simulink model "imageSendExample1"  (R2014a)
settings: configuration reference "AR_Drone_ConfigSet" (kept outside this file)
undefined symbols (not defined in the file): Afilter, Afilterphi, Amat, Bd, KDphi, KDphi_adjust, KDpsic, KDtheta, KDtheta_adjust, KDxc, KDyc, KDzc, KPphi, KPphi_adjust, KPpsic, KPtheta, KPtheta_adjust, KPxc, KPyc, KPzc, L, LA, LAphi, m
libraries: simulink x8, dspmtrx3 x5, AR_Drone_2_Library x4, ARdrone_video_lib x4, dspstat3 x2
(part 2 of 2)

== system imageSendExample1/Navigation Subsystem/CheckSum Pre-Processing/TempFilter/CheckSum Correction ==
  CalculatedData : Inport
  CheckSumFlag : Inport  Port=2
  Holding Value : Inport  Port=3
  Compare To Zero : simulink/Logic and Bit Operations/Compare To Zero  relop=>  OutDataTypeStr=boolean
  Delay : Delay  DelayLength=3  InitialCondition=0
  Generate Sample Holding Pulse : Subsystem
  "If True, we have good data, If false, we have bad data, With bad data, use previous good data from N samples ago and hold it on that value for M samples" : Switch  Criteria=u2 > Threshold
  Invert Logic : Logic  Operator=NOT  AllPortsSameDT=off  OutDataTypeStr=boolean
  Logical Operator1 : Logic  Operator=NOT  AllPortsSameDT=off  OutDataTypeStr=boolean
  Pre-Processed Data : Outport
  wires:
  CheckSumFlag/1 -> Compare To Zero/1
  CalculatedData/1 -> "If True, we have good data, If false, we have bad data, With bad data, use previous good data from N samples ago and hold it on that value for M samples"/1
  "If True, we have good data, If false, we have bad data, With bad data, use previous good data from N samples ago and hold it on that value for M samples"/1 -> Pre-Processed Data/1, Delay/1
  Delay/1 -> "If True, we have good data, If false, we have bad data, With bad data, use previous good data from N samples ago and hold it on that value for M samples"/3
  Compare To Zero/1 -> Logical Operator1/1
  Generate Sample Holding Pulse/1(Hold_Data_Pulse) -> Invert Logic/1
  Logical Operator1/1 -> Generate Sample Holding Pulse/1(CheckSumFlag)
  Invert Logic/1 -> "If True, we have good data, If false, we have bad data, With bad data, use previous good data from N samples ago and hold it on that value for M samples"/2
  Holding Value/1 -> Generate Sample Holding Pulse/2(HoldDataTicks_Value)

== system imageSendExample1/Navigation Subsystem/CheckSum Pre-Processing/TempFilter/Process Raw Mag Data ==
  note: magnetometer[ 0 ] = - ( float ) navdata.mx ;
      | magnetometer[ 1 ] = ( float ) navdata.my ;
      | magnetometer[ 2 ] = - ( float ) navdata.mz ;
      | const float Sensitivity[ 3 ] = { 0.0071492608 , 0.0070882491 , 0.0074057781 } ;
      | const float Neutral[ 3 ] = { 118.0 , - 65.0 , 110.0 } ;
  Magnetometer : Inport
  Bias : Constant  Value=[ 118.0, -65.0, 110.0 ]
  Sum : Sum  Inputs=|+-
  postGain : Gain  Gain=[0.0071492608, 0.0070882491, 0.0074057781]
  preGain : Gain  Gain=[-1 1 -1]
  ProcessedData : Outport
  wires:
  postGain/1 -> ProcessedData/1
  Magnetometer/1 -> preGain/1
  Sum/1 -> postGain/1
  preGain/1 -> Sum/1
  Bias/1 -> Sum/2

== system imageSendExample1/Navigation Subsystem/CheckSum Pre-Processing/TempFilter1/CheckSum Correction ==
  CalculatedData : Inport
  CheckSumFlag : Inport  Port=2
  Holding Value : Inport  Port=3
  Compare To Zero : simulink/Logic and Bit Operations/Compare To Zero  relop=>  OutDataTypeStr=boolean
  Delay : Delay  DelayLength=3  InitialCondition=0
  Generate Sample Holding Pulse : Subsystem
  "If True, we have good data, If false, we have bad data, With bad data, use previous good data from N samples ago and hold it on that value for M samples" : Switch  Criteria=u2 > Threshold
  Invert Logic : Logic  Operator=NOT  AllPortsSameDT=off  OutDataTypeStr=boolean
  Logical Operator1 : Logic  Operator=NOT  AllPortsSameDT=off  OutDataTypeStr=boolean
  Pre-Processed Data : Outport
  wires:
  CheckSumFlag/1 -> Compare To Zero/1
  CalculatedData/1 -> "If True, we have good data, If false, we have bad data, With bad data, use previous good data from N samples ago and hold it on that value for M samples"/1
  "If True, we have good data, If false, we have bad data, With bad data, use previous good data from N samples ago and hold it on that value for M samples"/1 -> Pre-Processed Data/1, Delay/1
  Delay/1 -> "If True, we have good data, If false, we have bad data, With bad data, use previous good data from N samples ago and hold it on that value for M samples"/3
  Compare To Zero/1 -> Logical Operator1/1
  Generate Sample Holding Pulse/1(Hold_Data_Pulse) -> Invert Logic/1
  Logical Operator1/1 -> Generate Sample Holding Pulse/1(CheckSumFlag)
  Invert Logic/1 -> "If True, we have good data, If false, we have bad data, With bad data, use previous good data from N samples ago and hold it on that value for M samples"/2
  Holding Value/1 -> Generate Sample Holding Pulse/2(HoldDataTicks_Value)

== system imageSendExample1/Navigation Subsystem/CheckSum Pre-Processing/TempFilter1/Process Raw Mag Data ==
  note: magnetometer[ 0 ] = - ( float ) navdata.mx ;
      | magnetometer[ 1 ] = ( float ) navdata.my ;
      | magnetometer[ 2 ] = - ( float ) navdata.mz ;
      | const float Sensitivity[ 3 ] = { 0.0071492608 , 0.0070882491 , 0.0074057781 } ;
      | const float Neutral[ 3 ] = { 118.0 , - 65.0 , 110.0 } ;
  Magnetometer : Inport
  Bias : Constant  Value=[ 118.0, -65.0, 110.0 ]
  Sum : Sum  Inputs=|+-
  postGain : Gain  Gain=[0.0071492608, 0.0070882491, 0.0074057781]
  preGain : Gain  Gain=[-1 1 -1]
  ProcessedData : Outport
  wires:
  postGain/1 -> ProcessedData/1
  Magnetometer/1 -> preGain/1
  Sum/1 -> postGain/1
  preGain/1 -> Sum/1
  Bias/1 -> Sum/2

== system imageSendExample1/Navigation Subsystem/CheckSum Pre-Processing/Ultrasound Processing/CheckSum Correction ==
  CalculatedData : Inport
  CheckSumFlag : Inport  Port=2
  Holding Value : Inport  Port=3
  Compare To Zero : simulink/Logic and Bit Operations/Compare To Zero  relop=>  OutDataTypeStr=boolean
  Delay : Delay  DelayLength=3  InitialCondition=0
  Generate Sample Holding Pulse : Subsystem
  "If True, we have good data, If false, we have bad data, With bad data, use previous good data from N samples ago and hold it on that value for M samples" : Switch  Criteria=u2 > Threshold
  Invert Logic : Logic  Operator=NOT  AllPortsSameDT=off  OutDataTypeStr=boolean
  Logical Operator1 : Logic  Operator=NOT  AllPortsSameDT=off  OutDataTypeStr=boolean
  Pre-Processed Height : Outport
  wires:
  CheckSumFlag/1 -> Compare To Zero/1
  CalculatedData/1 -> "If True, we have good data, If false, we have bad data, With bad data, use previous good data from N samples ago and hold it on that value for M samples"/1
  "If True, we have good data, If false, we have bad data, With bad data, use previous good data from N samples ago and hold it on that value for M samples"/1 -> Pre-Processed Height/1, Delay/1
  Delay/1 -> "If True, we have good data, If false, we have bad data, With bad data, use previous good data from N samples ago and hold it on that value for M samples"/3
  Compare To Zero/1 -> Logical Operator1/1
  Generate Sample Holding Pulse/1(Hold_Data_Pulse) -> Invert Logic/1
  Logical Operator1/1 -> Generate Sample Holding Pulse/1(CheckSumFlag)
  Invert Logic/1 -> "If True, we have good data, If false, we have bad data, With bad data, use previous good data from N samples ago and hold it on that value for M samples"/2
  Holding Value/1 -> Generate Sample Holding Pulse/2(HoldDataTicks_Value)

== system imageSendExample1/Navigation Subsystem/CheckSum Pre-Processing/Accelerometer Processing/CheckSum Correction/Generate Sample Holding Pulse ==
  CheckSumFlag : Inport
  HoldDataTicks_Value : Inport  Port=2
  Chart : Stateflow chart  TreatAsAtomicUnit=on
  Constant2 : Constant
  Logical Operator1 : Logic  AllPortsSameDT=off  OutDataTypeStr=boolean
  Transition Logic Detection : Subsystem
  Hold_Data_Pulse : Outport
  wires:
  Constant2/1 -> Logical Operator1/1
  Logical Operator1/1 -> Hold_Data_Pulse/1
  Chart/1(output) -> Logical Operator1/2
  Transition Logic Detection/1(Transition Detect) -> Chart/1(if_transition)
  CheckSumFlag/1 -> Transition Logic Detection/1(Input)
  HoldDataTicks_Value/1 -> Chart/2(HoldDataTicks)

== system imageSendExample1/Navigation Subsystem/CheckSum Pre-Processing/Magnetometer/CheckSum Correction/Generate Sample Holding Pulse ==
  CheckSumFlag : Inport
  HoldDataTicks_Value : Inport  Port=2
  Chart : Stateflow chart  TreatAsAtomicUnit=on
  Constant2 : Constant
  Logical Operator1 : Logic  AllPortsSameDT=off  OutDataTypeStr=boolean
  Transition Logic Detection : Subsystem
  Hold_Data_Pulse : Outport
  wires:
  Constant2/1 -> Logical Operator1/1
  Logical Operator1/1 -> Hold_Data_Pulse/1
  Chart/1(output) -> Logical Operator1/2
  Transition Logic Detection/1(Transition Detect) -> Chart/1(if_transition)
  CheckSumFlag/1 -> Transition Logic Detection/1(Input)
  HoldDataTicks_Value/1 -> Chart/2(HoldDataTicks)

== system imageSendExample1/Navigation Subsystem/CheckSum Pre-Processing/RateGyro Processing/CheckSum Correction/Generate Sample Holding Pulse ==
  CheckSumFlag : Inport
  HoldDataTicks_Value : Inport  Port=2
  Chart : Stateflow chart  TreatAsAtomicUnit=on
  Constant2 : Constant
  Logical Operator1 : Logic  AllPortsSameDT=off  OutDataTypeStr=boolean
  Transition Logic Detection : Subsystem
  Hold_Data_Pulse : Outport
  wires:
  Constant2/1 -> Logical Operator1/1
  Logical Operator1/1 -> Hold_Data_Pulse/1
  Chart/1(output) -> Logical Operator1/2
  Transition Logic Detection/1(Transition Detect) -> Chart/1(if_transition)
  CheckSumFlag/1 -> Transition Logic Detection/1(Input)
  HoldDataTicks_Value/1 -> Chart/2(HoldDataTicks)

== system imageSendExample1/Navigation Subsystem/CheckSum Pre-Processing/TempFilter/CheckSum Correction/Generate Sample Holding Pulse ==
  CheckSumFlag : Inport
  HoldDataTicks_Value : Inport  Port=2
  Chart : Stateflow chart  TreatAsAtomicUnit=on
  Constant2 : Constant
  Logical Operator1 : Logic  AllPortsSameDT=off  OutDataTypeStr=boolean
  Transition Logic Detection : Subsystem
  Hold_Data_Pulse : Outport
  wires:
  Constant2/1 -> Logical Operator1/1
  Logical Operator1/1 -> Hold_Data_Pulse/1
  Chart/1(output) -> Logical Operator1/2
  Transition Logic Detection/1(Transition Detect) -> Chart/1(if_transition)
  CheckSumFlag/1 -> Transition Logic Detection/1(Input)
  HoldDataTicks_Value/1 -> Chart/2(HoldDataTicks)

== system imageSendExample1/Navigation Subsystem/CheckSum Pre-Processing/TempFilter1/CheckSum Correction/Generate Sample Holding Pulse ==
  CheckSumFlag : Inport
  HoldDataTicks_Value : Inport  Port=2
  Chart : Stateflow chart  TreatAsAtomicUnit=on
  Constant2 : Constant
  Logical Operator1 : Logic  AllPortsSameDT=off  OutDataTypeStr=boolean
  Transition Logic Detection : Subsystem
  Hold_Data_Pulse : Outport
  wires:
  Constant2/1 -> Logical Operator1/1
  Logical Operator1/1 -> Hold_Data_Pulse/1
  Chart/1(output) -> Logical Operator1/2
  Transition Logic Detection/1(Transition Detect) -> Chart/1(if_transition)
  CheckSumFlag/1 -> Transition Logic Detection/1(Input)
  HoldDataTicks_Value/1 -> Chart/2(HoldDataTicks)

== system imageSendExample1/Navigation Subsystem/CheckSum Pre-Processing/Ultrasound Processing/CheckSum Correction/Generate Sample Holding Pulse ==
  CheckSumFlag : Inport
  HoldDataTicks_Value : Inport  Port=2
  Chart : Stateflow chart  TreatAsAtomicUnit=on
  Constant2 : Constant
  Logical Operator1 : Logic  AllPortsSameDT=off  OutDataTypeStr=boolean
  Transition Logic Detection : Subsystem
  Hold_Data_Pulse : Outport
  wires:
  Constant2/1 -> Logical Operator1/1
  Logical Operator1/1 -> Hold_Data_Pulse/1
  Chart/1(output) -> Logical Operator1/2
  Transition Logic Detection/1(Transition Detect) -> Chart/1(if_transition)
  CheckSumFlag/1 -> Transition Logic Detection/1(Input)
  HoldDataTicks_Value/1 -> Chart/2(HoldDataTicks)

== system imageSendExample1/Navigation Subsystem/CheckSum Pre-Processing/Accelerometer Processing/CheckSum Correction/Generate Sample Holding Pulse/Transition Logic Detection ==
  Input : Inport
  Constant : Constant  Value=0
  Constant1 : Constant
  Logical Operator : Logic  AllPortsSameDT=off  OutDataTypeStr=boolean
  Relational Operator : RelationalOperator  Operator===  OutDataTypeStr=boolean
  Relational Operator1 : RelationalOperator  Operator===  OutDataTypeStr=boolean
  Unit Delay : UnitDelay  SampleTime=-1
  Transition Detect : Outport
  wires:
  Relational Operator1/1 -> Logical Operator/1
  Unit Delay/1 -> Relational Operator/1
  Input/1 -> Relational Operator1/2, Unit Delay/1
  Relational Operator/1 -> Logical Operator/2
  Constant/1 -> Relational Operator/2
  Constant1/1 -> Relational Operator1/1
  Logical Operator/1 -> Transition Detect/1  "Transition_Detect"

== system imageSendExample1/Navigation Subsystem/CheckSum Pre-Processing/Magnetometer/CheckSum Correction/Generate Sample Holding Pulse/Transition Logic Detection ==
  Input : Inport
  Constant : Constant  Value=0
  Constant1 : Constant
  Logical Operator : Logic  AllPortsSameDT=off  OutDataTypeStr=boolean
  Relational Operator : RelationalOperator  Operator===  OutDataTypeStr=boolean
  Relational Operator1 : RelationalOperator  Operator===  OutDataTypeStr=boolean
  Unit Delay : UnitDelay  SampleTime=-1
  Transition Detect : Outport
  wires:
  Relational Operator1/1 -> Logical Operator/1
  Unit Delay/1 -> Relational Operator/1
  Input/1 -> Relational Operator1/2, Unit Delay/1
  Relational Operator/1 -> Logical Operator/2
  Constant/1 -> Relational Operator/2
  Constant1/1 -> Relational Operator1/1
  Logical Operator/1 -> Transition Detect/1  "Transition_Detect"

== system imageSendExample1/Navigation Subsystem/CheckSum Pre-Processing/RateGyro Processing/CheckSum Correction/Generate Sample Holding Pulse/Transition Logic Detection ==
  Input : Inport
  Constant : Constant  Value=0
  Constant1 : Constant
  Logical Operator : Logic  AllPortsSameDT=off  OutDataTypeStr=boolean
  Relational Operator : RelationalOperator  Operator===  OutDataTypeStr=boolean
  Relational Operator1 : RelationalOperator  Operator===  OutDataTypeStr=boolean
  Unit Delay : UnitDelay  SampleTime=-1
  Transition Detect : Outport
  wires:
  Relational Operator1/1 -> Logical Operator/1
  Unit Delay/1 -> Relational Operator/1
  Input/1 -> Relational Operator1/2, Unit Delay/1
  Relational Operator/1 -> Logical Operator/2
  Constant/1 -> Relational Operator/2
  Constant1/1 -> Relational Operator1/1
  Logical Operator/1 -> Transition Detect/1  "Transition_Detect"

== system imageSendExample1/Navigation Subsystem/CheckSum Pre-Processing/TempFilter/CheckSum Correction/Generate Sample Holding Pulse/Transition Logic Detection ==
  Input : Inport
  Constant : Constant  Value=0
  Constant1 : Constant
  Logical Operator : Logic  AllPortsSameDT=off  OutDataTypeStr=boolean
  Relational Operator : RelationalOperator  Operator===  OutDataTypeStr=boolean
  Relational Operator1 : RelationalOperator  Operator===  OutDataTypeStr=boolean
  Unit Delay : UnitDelay  SampleTime=-1
  Transition Detect : Outport
  wires:
  Relational Operator1/1 -> Logical Operator/1
  Unit Delay/1 -> Relational Operator/1
  Input/1 -> Relational Operator1/2, Unit Delay/1
  Relational Operator/1 -> Logical Operator/2
  Constant/1 -> Relational Operator/2
  Constant1/1 -> Relational Operator1/1
  Logical Operator/1 -> Transition Detect/1  "Transition_Detect"

== system imageSendExample1/Navigation Subsystem/CheckSum Pre-Processing/TempFilter1/CheckSum Correction/Generate Sample Holding Pulse/Transition Logic Detection ==
  Input : Inport
  Constant : Constant  Value=0
  Constant1 : Constant
  Logical Operator : Logic  AllPortsSameDT=off  OutDataTypeStr=boolean
  Relational Operator : RelationalOperator  Operator===  OutDataTypeStr=boolean
  Relational Operator1 : RelationalOperator  Operator===  OutDataTypeStr=boolean
  Unit Delay : UnitDelay  SampleTime=-1
  Transition Detect : Outport
  wires:
  Relational Operator1/1 -> Logical Operator/1
  Unit Delay/1 -> Relational Operator/1
  Input/1 -> Relational Operator1/2, Unit Delay/1
  Relational Operator/1 -> Logical Operator/2
  Constant/1 -> Relational Operator/2
  Constant1/1 -> Relational Operator1/1
  Logical Operator/1 -> Transition Detect/1  "Transition_Detect"

== system imageSendExample1/Navigation Subsystem/CheckSum Pre-Processing/Ultrasound Processing/CheckSum Correction/Generate Sample Holding Pulse/Transition Logic Detection ==
  Input : Inport
  Constant : Constant  Value=0
  Constant1 : Constant
  Logical Operator : Logic  AllPortsSameDT=off  OutDataTypeStr=boolean
  Relational Operator : RelationalOperator  Operator===  OutDataTypeStr=boolean
  Relational Operator1 : RelationalOperator  Operator===  OutDataTypeStr=boolean
  Unit Delay : UnitDelay  SampleTime=-1
  Transition Detect : Outport
  wires:
  Relational Operator1/1 -> Logical Operator/1
  Unit Delay/1 -> Relational Operator/1
  Input/1 -> Relational Operator1/2, Unit Delay/1
  Relational Operator/1 -> Logical Operator/2
  Constant/1 -> Relational Operator/2
  Constant1/1 -> Relational Operator1/1
  Logical Operator/1 -> Transition Detect/1  "Transition_Detect"

== stateflow chart imageSendExample1/Navigation Subsystem/CheckSum Pre-Processing/Accelerometer Processing/CheckSum Correction/Generate Sample Holding Pulse/Chart ==
  state Begin_State0
    entry: output =0;
  state Begin_State
    entry: output =1;
  state End_State
    entry: output=0;
  (default) -> Begin_State0
  Begin_State0 -> Begin_State : [if_transition==1]
  Begin_State -> End_State [order 1] : after(HoldDataTicks,tick)
  End_State -> Begin_State : [if_transition==1]
  Begin_State -> Begin_State [order 2] : [if_transition==1]
  data: output output; if_transition input; HoldDataTicks input

== stateflow chart imageSendExample1/Navigation Subsystem/CheckSum Pre-Processing/Magnetometer/CheckSum Correction/Generate Sample Holding Pulse/Chart ==
  state Begin_State0
    entry: output =0;
  state Begin_State
    entry: output =1;
  state End_State
    entry: output=0;
  (default) -> Begin_State0
  Begin_State0 -> Begin_State : [if_transition==1]
  Begin_State -> End_State [order 1] : after(HoldDataTicks,tick)
  End_State -> Begin_State : [if_transition==1]
  Begin_State -> Begin_State [order 2] : [if_transition==1]
  data: output output; if_transition input; HoldDataTicks input

== stateflow chart imageSendExample1/Navigation Subsystem/CheckSum Pre-Processing/RateGyro Processing/CheckSum Correction/Generate Sample Holding Pulse/Chart ==
  state Begin_State0
    entry: output =0;
  state Begin_State
    entry: output =1;
  state End_State
    entry: output=0;
  (default) -> Begin_State0
  Begin_State0 -> Begin_State : [if_transition==1]
  Begin_State -> End_State [order 1] : after(HoldDataTicks,tick)
  End_State -> Begin_State : [if_transition==1]
  Begin_State -> Begin_State [order 2] : [if_transition==1]
  data: output output; if_transition input; HoldDataTicks input

== stateflow chart imageSendExample1/Navigation Subsystem/CheckSum Pre-Processing/TempFilter/CheckSum Correction/Generate Sample Holding Pulse/Chart ==
  state Begin_State0
    entry: output =0;
  state Begin_State
    entry: output =1;
  state End_State
    entry: output=0;
  (default) -> Begin_State0
  Begin_State0 -> Begin_State : [if_transition==1]
  Begin_State -> End_State [order 1] : after(HoldDataTicks,tick)
  End_State -> Begin_State : [if_transition==1]
  Begin_State -> Begin_State [order 2] : [if_transition==1]
  data: output output; if_transition input; HoldDataTicks input

== stateflow chart imageSendExample1/Navigation Subsystem/CheckSum Pre-Processing/TempFilter1/CheckSum Correction/Generate Sample Holding Pulse/Chart ==
  state Begin_State0
    entry: output =0;
  state Begin_State
    entry: output =1;
  state End_State
    entry: output=0;
  (default) -> Begin_State0
  Begin_State0 -> Begin_State : [if_transition==1]
  Begin_State -> End_State [order 1] : after(HoldDataTicks,tick)
  End_State -> Begin_State : [if_transition==1]
  Begin_State -> Begin_State [order 2] : [if_transition==1]
  data: output output; if_transition input; HoldDataTicks input

== stateflow chart imageSendExample1/Navigation Subsystem/CheckSum Pre-Processing/Ultrasound Processing/CheckSum Correction/Generate Sample Holding Pulse/Chart ==
  state Begin_State0
    entry: output =0;
  state Begin_State
    entry: output =1;
  state End_State
    entry: output=0;
  (default) -> Begin_State0
  Begin_State0 -> Begin_State : [if_transition==1]
  Begin_State -> End_State [order 1] : after(HoldDataTicks,tick)
  End_State -> Begin_State : [if_transition==1]
  Begin_State -> Begin_State [order 2] : [if_transition==1]
  data: output output; if_transition input; HoldDataTicks input

== matlab function imageSendExample1/Controller/Conversion torques to motor speeds/MATLAB Function ==
  data: u input; y output
function y = forcestorques2motorspeeds(u)
% static transformation

% inverse of transformation 

% inv([1 1 1 1; 1 -1 -1 1; 1 1 -1 -1;-1 1 -1 1]) = 
% 1/4*[1 1 1 -1; 1  -1  1  1; 1 -1 -1 -1; 1  1 -1  1]

% L = 0.1785, L*sqrt(2)/2 = 0.1262, 1/(L*sqrt(2)/2) = 7.9228
% CM = 0.025; 1/CM = 40;

forcestorques = u;

% saturations -------------------------------------------------------------

% saturate total thrust
if forcestorques(1) > 7.2 % 1.8*4 = 7.2 max torque of each propeller determined experimentally
    forcestorques(1) = 7.2;
elseif forcestorques(1) < 0.56 % 0.14*4 = 0.56 min torque of each propeller determined experimentally
    forcestorques(1) = 0.56;
end

% saturate moments

CM = 0.025;
% compute max abs torque for a worst case situation
maxabstorque1 = (7.2-forcestorques(1))/(3*7.9228);
maxabstorque2 = (forcestorques(1)-0.56)/(3*7.9228);
maxabstorque = min(maxabstorque1,maxabstorque2);
maxabstorquepsi = maxabstorque*7.9228*CM;
if forcestorques(2) > maxabstorque
    forcestorques(2) = maxabstorque;
elseif forcestorques(2) < -maxabstorque
    forcestorques(2) = -maxabstorque;
end

if forcestorques(3) > maxabstorque
    forcestorques(3) = maxabstorque;
elseif forcestorques(3) < -maxabstorque
    forcestorques(3) = -maxabstorque;
end

if forcestorques(4) >maxabstorquepsi
    forcestorques(4) = maxabstorquepsi
elseif forcestorques(4) < -maxabstorquepsi
    forcestorques(4) = -maxabstorquepsi;
end
%  ------------------------------------------------------------------------



AA = [1.0000    1.0000    1.0000   -1.0000
    1.0000   -1.0000    1.0000    1.0000
    1.0000   -1.0000   -1.0000   -1.0000
    1.0000    1.0000   -1.0000    1.0000];

forcespropellers=  1/4*AA*diag([1 7.9228 7.9228 1/CM])*forcestorques;


 % invert function determined experimentally see ActuationThrustFit
 a = 0.135415000000000;
 b = 0.006931357945865;
 c = 1.487800000000000e-04;
 
 motorspeeds = floor( (-b + sqrt( b^2 - 4*(a-forcespropellers)*c ))/(2*c));
 
y = motorspeeds;

== matlab function imageSendExample1/Navigation Subsystem/CheckSum Pre-Processing/Ultrasound Processing/Height Calculation ==
  data: u input double; y output double; prev_good_height output double; z_1 input double
function [y,prev_good_height] = fcn(u,z_1)
%#codegen



if u<10000
    
    height = ((u - 880) /26.553);
    prev_good_height = height;
else
    
%     height = u;
%     prev_good_height = height;
    height =  z_1;
    prev_good_height = z_1; 
end

y = height;

== stateflow chart imageSendExample1/Control State Chart/Supervisory Flight Controller ==
  state Fault_Check [parallel]
    settings: executionOrder=4
    state BatteryFault_Check [parallel]
      settings: executionOrder=1
      state BatteryNominal
        en:
        BatteryFault = 0;
        state Nominal
        note: Description:
            | This state will be responsible for the following
            |
            | - Automatically land the drone by forcing it to the land state when voltage is low
            | - Prevent drone from taking off if battery voltage is too low
        state EvaluateVoltageLevel
        state ChangeState
          en:
          BatteryFault = 1;
        EvaluateVoltageLevel -> Nominal [order 1] : [Measured_Battery_Voltage>=10.1]
        Nominal -> EvaluateVoltageLevel : [Measured_Battery_Voltage<10.1]
        (default) -> EvaluateVoltageLevel
        EvaluateVoltageLevel -> ChangeState [order 2] : after(5,sec)
      state BatteryLow
        state ForceLanding
          en:
        (default) -> ForceLanding
      (default) -> BatteryNominal
    state UltraSoundwarning_Check [parallel]
      settings: executionOrder=2
    state SafeOrientation_Check [parallel]
      settings: executionOrder=3
      state UnsafeOrientation
        du:
        MotorArmed =0;
        LandingPhase = 0;
      state WaitForFlight
      state GravityVectorCheck
        en:
        OrientationFault = 0;
        note: ALAWAYS IN SAFE MODE
      (default) -> WaitForFlight
      GravityVectorCheck -> WaitForFlight : [in(Drone_State.WaitForHost)]
      WaitForFlight -> GravityVectorCheck : [in(Drone_State.Controlled_Flight)]
  state Drone_State [parallel]
    settings: executionOrder=1
    state WaitForHost
      entry:
      reset_offset_calc = 0;
      MotorArmed = 0;
      MotorArmedInitialize =0;
      LandingProperly =0;
      refHeight = 0;
      LandingPhase = 0;
      initDone=0;
    state Calibration
      entry:
      reset_calib=1;
      quadOr = 0;
      state gyro = calibGyro(signal,reset) [function]
      state [min,avg,max] = calibAccel(signal,reset) [function]
      state calibAccelRunning [parallel]
        entry,during:[accelMin, accelAvg, accelMax] =calibAccel(accel, reset_calib);
        settings: executionOrder=4
      state calibGyroRunnning [parallel]
        entry,during:gyroTemp=calibGyro(gyro,reset_calib)
        settings: executionOrder=1
      state Gyro1 [parallel]
        settings: executionOrder=2
        state Nothing
        state Read
          entry:
          reset_calib=0;
        state Write
          entry:
          gyro_offset= -gyroTemp';
        state noop4
        (default) -> Nothing
        Nothing -> Drone_State.Calibration.Gyro1.Read : [quadOr ==2]
        Drone_State.Calibration.Gyro1.Read -> Write : [after(4,sec)]
        Write -> noop4 : [after(.5,sec)]
      state Accel1 [parallel]
        settings: executionOrder=5
        state Read
          entry:
          reset_calib=0;
        state noop
        state noop1
        state Write1
          entry:accel_temp_mat(3,1)= accelMin(3);
          accel_temp_mat(1,2)= accelAvg(1);
          accel_temp_mat(2,2)= accelAvg(2);
        state Write2
          entry:accel_temp_mat(3,3)= accelMax(3);
          accel_temp_mat(1,2)= accelAvg(1);
          accel_temp_mat(2,2)= accelAvg(2);
        state Write3
          entry:accel_temp_mat(2,1)= accelMin(2);
          accel_temp_mat(1,2)= accelAvg(1);
          accel_temp_mat(3,2)= accelAvg(3);
        state Write4
          entry:accel_temp_mat(2,3)= accelMax(2);
          accel_temp_mat(1,2)= accelAvg(1);
          accel_temp_mat(3,2)= accelAvg(3);
        state Write5
          entry:accel_temp_mat(1,1)= accelMin(1);
          accel_temp_mat(2,2)= accelAvg(2);
          accel_temp_mat(3,2)=accelAvg(3);
        state Write6
          entry:accel_temp_mat(1,3)= accelMax(1);
          accel_temp_mat(2,2)= accelAvg(2);
          accel_temp_mat(3,2)= accelAvg(3);
        state noop3
        noop1 -> Drone_State.Calibration.Accel1.Read : [quadOr~=0]
        noop -> Write5 [order 5] : [quadOr==5]
        Drone_State.Calibration.Accel1.Read -> noop : after(4,sec)
        noop -> Write6 [order 6] : [quadOr==6]
        noop -> Write4 [order 4] : [quadOr==4]
        noop -> Write3 [order 3] : [quadOr==3]
        noop -> Write2 [order 2] : [quadOr==2]
        noop -> Write1 [order 1] : [quadOr==1]
        Write1 -> noop3 : after(.5,sec)
        (default) -> noop1
        Write2 -> noop3 : after(.5,sec)
        Write3 -> noop3 : after(.5,sec)
        Write4 -> noop3 : after(.5,sec)
        Write5 -> noop3 : after(.5,sec)
        Write6 -> noop3 : after(.5,sec)
      state quad_orient = getPosition(accel) [function]
      state Position [parallel]
        entry: quadOr = getPosition(accel);
        during: reset_calib=0; quadOr = getPosition(accel);
        settings: executionOrder=3
    state Take_offsequence
      entry:
      LandingPhase = 0;
      refHeight = 0;
      MotorArmedInitialize =1;
      LandingProperly =0;
      MotorArmed = 0;
      state PM_5
        entry:
        c_1 = 20;
        c_2 = 20;
        c_3 = 20;
        c_4 =20;
      state Done_Initialization
        entry:
      state PMW
        entry:
        c_1 = 40;
        c_2 = 40;
        c_3 = 40;
        c_4 = 40;
      (default) -> PM_5
      PM_5 -> Drone_State.Take_offsequence.PMW : [after(2,sec)]
      Drone_State.Take_offsequence.PMW -> Drone_State.Take_offsequence.Done_Initialization
    state Controlled_Flight
      entry:
      LandingPhase = 0;
      refHeight = 0;
      MotorArmed =1;
      MotorArmedInitialize =0;
      note: 
      state nothing
        entry:KDC=0.5
        T=0
        P=0
      note: KDC IS THE HEIGHT INPUT THAT GOES TO THE REFERENCE BLOCK
          | VALUES T and P CAN BE USED TO DEFINE ANY OTHER SUCH STATE,
          | AT PRESENT T and P ARE NOT USED ANYWHERE
      state change
        entry:KDC=1
        T=0
        P=0
      state change1
        entry:KDC=1
        T=0
        P=0
      state change2
        entry:KDC=1.5
        T=1
        P=1
      state change3
        entry:KDC=2
      state change4
        entry:KDC=2
      note: ?
      (default) -> nothing
      nothing -> change : after(1,sec)
      change -> change1 : after(3,sec)
      change1 -> change2 : after(3,sec)
      change3 -> change4 : after(1,sec)
      change2 -> change3 : after(3,sec)
    state Landing_Sequence
      entry:
      LandingProperly =1;
      LandingPhase = 0; refHeight = 0; MotorArmed =0; MotorArmedInitialize =0;
      state PMW
        entry:
        a1 = 60;
        a2 =60;
        a3 = 60;;
        a4 = 60;
      state PMW_15
        entry:
        a1 = 0;
        a2 = 0;
        a3 = 0;
        a4 = 0;
      state Done_Initialization
        entry:
      state PMW_30
        entry:
        a1 =50;
        a2 = 50;
        a3 = 50;
        a4 = 50;
      state PMW_25
        entry:
        a1 = 20;
        a2 = 20;
        a3 = 20;
        a4 = 20;
      (default) -> Drone_State.Landing_Sequence.PMW [order 1]
      (default) -> Drone_State.Landing_Sequence.PMW [order 2]
      Drone_State.Landing_Sequence.PMW -> PMW_30 : [after(2,sec)]
      PMW_25 -> PMW_15 : [after(2,sec)]
      PMW_15 -> Drone_State.Landing_Sequence.Done_Initialization
      PMW_30 -> PMW_25 : [after(2,sec)]
    state Landing_Terminate
      entry:
      MotorArmed =0;
      MotorArmedInitialize =0;
      LandingPhase = 1;
    (default) -> WaitForHost
    Landing_Terminate -> WaitForHost
    WaitForHost -> Calibration [order 2] : [ hostCmd ==1 ]
    Calibration -> WaitForHost [order 2] : [hostCmd == 0]
    WaitForHost -> Take_offsequence [order 1] : [ hostCmd == 2 ]
    Calibration -> Take_offsequence [order 1] : [ hostCmd ==2 ]
    Take_offsequence -> Landing_Sequence [order 2] : [hostCmd ==3]
    Take_offsequence -> Controlled_Flight [order 1] : [ hostCmd == 4 ]
    Controlled_Flight -> Landing_Terminate [order 2] : [altitude == 2]
    Controlled_Flight -> Landing_Sequence [order 1] : [hostCmd ==3]
    Landing_Sequence -> Landing_Terminate : after(5,sec)
  state motor_landing [parallel]
    entry,during:
    MotorCMD=func(c1,c2,c3,c4,LandingPhase,MotorArmed,MotorArmedInitialize,c_1,c_2,c_3,c_4,a1,a2,a3,a4,LandingProperly)
    settings: executionOrder=3
  state Mcommands = func(c_a1,c_a2,c_a3,c_a4,Landing_Phase,Motor_Armed,MotorArmed_Initialize,cz1,cz2,cz3,cz4,a_1,a_2,a_3,a_4,Landing_Properly) [function]
  state ou [parallel]
    entry,during:
    outp=MotorCMD
    settings: executionOrder=2
  data: signal function_input double size=3; gyro function_output; reset function_input double size=1; min function_output; avg function_output; max function_output; signal function_input double size=3; reset function_input double size=1; accel function_input double size=3; quad_orient function_output double size=1; Mcommands function_output; c_a1 function_input double size=1; c_a2 function_input double size=1; c_a3 function_input double size=1; c_a4 function_input double size=1; Landing_Phase function_input double size=1; Motor_Armed function_input double size=1; MotorArmed_Initialize function_input double size=1; cz1 function_input double size=1; cz2 function_input double size=1; cz3 function_input double size=1; cz4 function_input double size=1; a_1 function_input double size=1; a_2 function_input double size=1; a_3 function_input double size=1; a_4 function_input double size=1; Landing_Properly function_input double size=1; hostCmd input double; initDone local; throttle local int16; height local; hoverHeight local; Measured_Battery_Voltage input; Converge_Flag local; reset_offset_calc local; MotorArmed local; LandingPhase local; N local; Offset_Parameters input size=2; GyroOffset_Parameters input size=3; BatteryFault local; OrientationFault local; refHeight output; UltraSound_Feedback input; NominalThrust local; MotorCMD local; outp output; c1 input; c2 input; c3 input; c4 input; altitude input double; Desired_Altitude local; a3 local; a4 local; a1 local; a2 local; MotorArmedInitialize local; LandingProperly local; c_1 output; c_2 output; c_4 output; c_3 output; KDC data_store_memory; XC input; YC input; y input; x input; P data_store_memory; T data_store_memory; accel input; gyro input; gyro_offset data_store_memory; accel_temp_mat data_store_memory; quadOr local; gyroTemp local; reset_calib local; accelMin local; accelAvg local; accelMax local
  data hostCmd settings: description=|
      | The hostCmd can take the values 0,1 and 2.
      | 
      | 0 - default state when the drone is powered up.
      | 1 - Takeoff
      | 2 - Landing
  data initDone settings: description=A flag to check whether the calibration is done.
  data refHeight settings: description=Desired height at which the drone needs to hover.
